simulink model "Pacemaker_Group1_1"  (R2020a)
settings: Solver=FixedStepAuto  StartTime=0.0  StopTime=10.0  FixedStep=1e-3  RelTol=1e-3  EnableMultiTasking=on
undefined symbols (not defined in the file): D0, D1, D10, D11, D12, D13, D2, D3, D4, D5, D6, D7, D8, D9, PTA0, PTA1, PTA2, PTB23, PTB9, PTC16, PTC17, PTC2, PTC3, PTC4, PTD0, PTD1, PTD2, PTD3
libraries: frdmk64flib x17
settings Model: SimulationMode=external  ExtModeTrigDuration=5  Creator=Luis  LastModifiedBy=jordanbierbrier
settings OptimizationCC: EnhancedBackFolding=on  PassReuseOutputArgsAs=Individual arguments  ZeroExternalMemoryAtStartup=off  ZeroInternalMemoryAtStartup=off  MaxStackSize=64  OptimizeBlockOrder=speed  DifferentSizesBufferReuse=on  OptimizationCustomize=off  EfficientTunableParamExpr=on
settings DebuggingCC: ParameterTunabilityLossMsg=error
settings HardwareCC: ProdBitPerPointer=32  ProdBitPerSizeT=32  ProdBitPerPtrDiffT=32  ProdLargestAtomicInteger=Long  ProdLargestAtomicFloat=Double  ProdWordSize=32  ProdHWDeviceType=ARM Compatible->ARM Cortex
settings SFSimCC: MATLABDynamicMemAlloc=off
settings RTWCC: SystemTargetFile=ert.tlc  HardwareBoard=NXP FRDM-K64F  TemplateMakefile=ert_default_tmf  Toolchain=GNU Tools for ARM Embedded Processors
settings CodeAppCC: ForceParamTrailComments=on  IgnoreCustomStorageClasses=off  OperatorAnnotations=on  SimulinkDataObjDesc=on  SFDataObjDesc=on  InsertBlockDesc=on
settings ERTTargetCC: ExtMode=on  ExtModeTransport=4  ExtModeMexFile=sendToCommService  ExtModeMexArgs='Pacemaker_Group1' 0

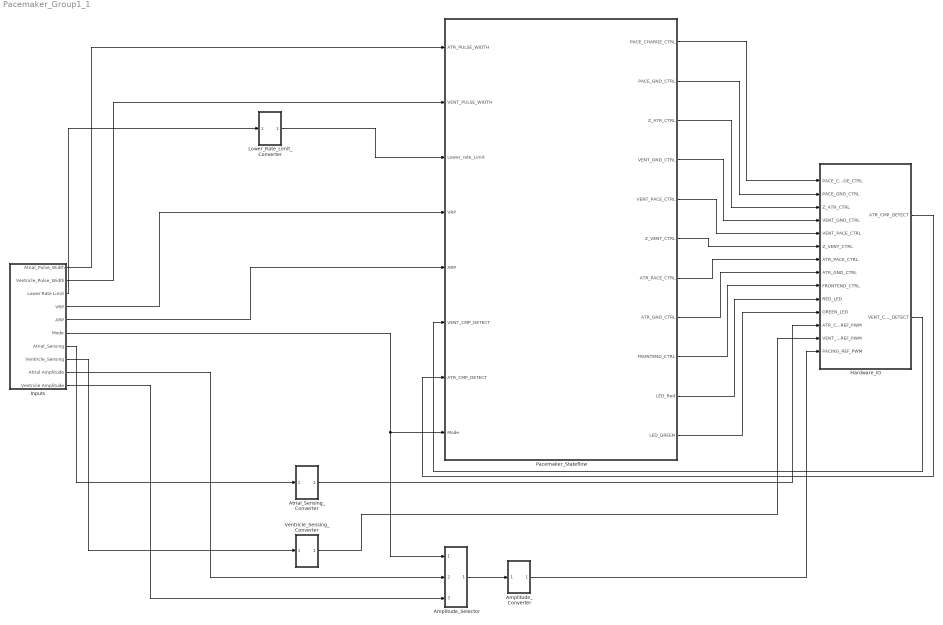
== system Pacemaker_Group1_1 ==
  Amplitude_Converter : Subsystem
  Amplitude_Selector : Subsystem
  Atrial_Sensing_Converter : Subsystem
  Hardware_IO : Subsystem
  Inputs : Subsystem
  Lower_Rate_Limit_Converter : Subsystem
  "Pacemaker_Stateflow " : Stateflow chart  TreatAsAtomicUnit=on
      settings: PortSchema="{\"entries\":[{\"content\":{\"sides\":[{\"content\":{\"connectorIds\":[\"In1\",\"In4\",\"In2\",\"In5\",\"In6\",\"In7\",\"In8\",\"In3\"]},\"type\":\"ConnectorPlacement.EquallySpacedRectSide\",\"uuid\":\"f97b12ff-cb00-4386-a373-7143c3a8b48d\"},{\"content\":{\"connectorIds\":[\"Out1\",\"Out2\",\"Out3\",\"Out4\",\"Out5\",\"Out6\",\"Out7\",\"Out8\",\"Out9\",\"Out10\",\"Out11\"],\"side\":\"RIGHT\"},\"type\":\"ConnectorPlacement.EquallySpacedRectSide\",\"uuid\":\"90163773-f9d1-46de-bd72-9589b8539202\"},{\"content\":{\"connectorIds\":[],\"side\":\"TOP\"},\"type\":\"ConnectorPlacement.EquallySpacedRectSide\",\"uuid\":\"f8a54119-a7c4-4071-8260-df405210e670\"},{\"content\":{\"connectorIds\":[],\"side\":\"BOTTOM\"},\"type\":\"ConnectorPlacement.EquallySpacedRectSide\",\"uuid\":\"70f9d800-d0b8-46e1-812e-9f4712f7acbd\"}]},\"type\":\"ConnectorPlacement.EquallySpacedConnector\",\"uuid\":\"47f7c40c-c42b-42f7-beed-99d299c6cdee\"}],\"packageUris\":[\"http://schema.mathworks.com/mf0/Connector/19700101\"],\"version\":\"1.0\"}"
  Ventricle_Sensing_Converter : Subsystem
  wires:
  Lower_Rate_Limit_Converter/1(Out1) -> "Pacemaker_Stateflow "/2(Lower_rate_Limit)
  Amplitude_Selector/1(Out1) -> Amplitude_Converter/1(In1)
  "Pacemaker_Stateflow "/1(PACE_CHARGE_CTRL) -> Hardware_IO/1(PACE_CHARGE_CTRL)
  "Pacemaker_Stateflow "/2(PACE_GND_CTRL) -> Hardware_IO/2(PACE_GND_CTRL)
  "Pacemaker_Stateflow "/3(Z_ATR_CTRL) -> Hardware_IO/3(Z_ATR_CTRL)
  "Pacemaker_Stateflow "/4(VENT_GND_CTRL) -> Hardware_IO/4(VENT_GND_CTRL)
  "Pacemaker_Stateflow "/5(VENT_PACE_CTRL) -> Hardware_IO/5(VENT_PACE_CTRL)
  "Pacemaker_Stateflow "/6(Z_VENT_CTRL) -> Hardware_IO/6(Z_VENT_CTRL)
  "Pacemaker_Stateflow "/7(ATR_PACE_CTRL) -> Hardware_IO/7(ATR_PACE_CTRL)
  "Pacemaker_Stateflow "/8(ATR_GND_CTRL) -> Hardware_IO/8(ATR_GND_CTRL)
  "Pacemaker_Stateflow "/9(FRONTEND_CTRL) -> Hardware_IO/9(FRONTEND_CTRL)
  "Pacemaker_Stateflow "/10(LED_Red) -> Hardware_IO/10(RED_LED)
  "Pacemaker_Stateflow "/11(LED_GREEN) -> Hardware_IO/11(GREEN_LED)
  Ventricle_Sensing_Converter/1(Out1) -> Hardware_IO/13(VENT_CMP_REF_PWM)
  Amplitude_Converter/1(Out1) -> Hardware_IO/14(PACING_REF_PWM)
  Hardware_IO/1(ATR_CMP_DETECT) -> "Pacemaker_Stateflow "/8(ATR_CMP_DETECT)
  Hardware_IO/2(VENT_CMP_DETECT) -> "Pacemaker_Stateflow "/7(VENT_CMP_DETECT)
  Atrial_Sensing_Converter/1(Out1) -> Hardware_IO/12(ATR_CMP_REF_PWM)
  Inputs/6(Mode) -> Amplitude_Selector/1(In1), "Pacemaker_Stateflow "/3(Mode)
  Inputs/1(Atrial_Pulse_Width) -> "Pacemaker_Stateflow "/1(ATR_PULSE_WIDTH)
  Inputs/2(Ventricle_Pulse_Width) -> "Pacemaker_Stateflow "/4(VENT_PULSE_WIDTH)
  Inputs/3(Lower Rate Limit) -> Lower_Rate_Limit_Converter/1(In1)
  Inputs/4(VRP) -> "Pacemaker_Stateflow "/5(VRP)
  Inputs/5(ARP) -> "Pacemaker_Stateflow "/6(ARP)
  Inputs/7(Atrial_Sensing) -> Atrial_Sensing_Converter/1(In1)
  Inputs/8(Ventricle_Sensing) -> Ventricle_Sensing_Converter/1(In1)
  Inputs/9(Atrial Amplitude) -> Amplitude_Selector/2(In2)
  Inputs/10(Ventricle Amplitude) -> Amplitude_Selector/3(In3)

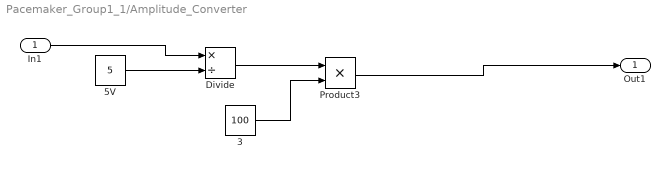
== system Pacemaker_Group1_1/Amplitude_Converter ==
  In1 : Inport
  3 : Constant  Value=100  OutDataTypeStr=double
  5V : Constant  Value=5  OutDataTypeStr=double
  Divide : Product  Inputs=*/  OutDataTypeStr=double  RndMeth=Nearest
  Product3 : Product  OutDataTypeStr=double
  Out1 : Outport
  wires:
  Product3/1 -> Out1/1
  3/1 -> Product3/2
  In1/1 -> Divide/1
  Divide/1 -> Product3/1
  5V/1 -> Divide/2

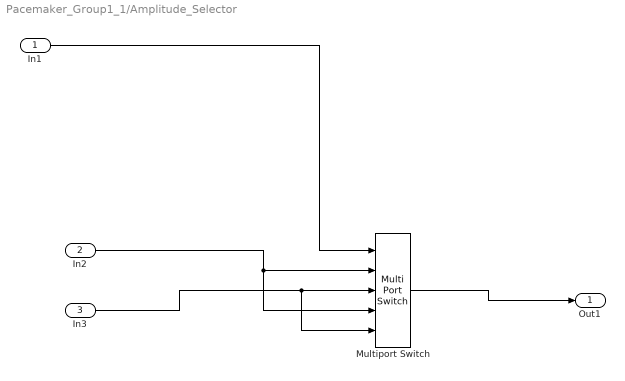
== system Pacemaker_Group1_1/Amplitude_Selector ==
  In1 : Inport
  In2 : Inport  Port=2
  In3 : Inport  Port=3
  Multiport Switch : MultiPortSwitch  DataPortOrder=Zero-based contiguous  Inputs=4  zeroidx=on  OutDataTypeStr=double
  Out1 : Outport
  wires:
  Multiport Switch/1 -> Out1/1
  In3/1 -> Multiport Switch/5, Multiport Switch/3
  In1/1 -> Multiport Switch/1
  In2/1 -> Multiport Switch/4, Multiport Switch/2

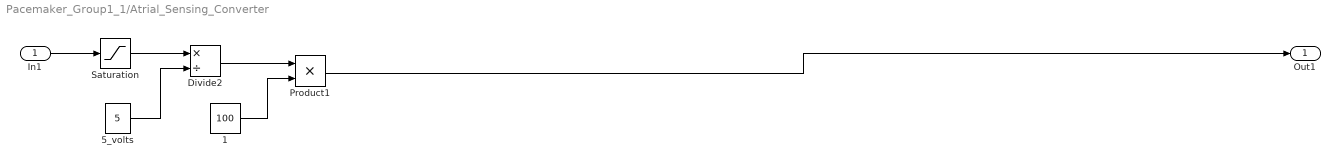
== system Pacemaker_Group1_1/Atrial_Sensing_Converter ==
  In1 : Inport
  1 : Constant  Value=100  OutDataTypeStr=uint16
  5_volts : Constant  Value=5  OutDataTypeStr=double
  Divide2 : Product  Inputs=*/
  Product1 : Product  OutDataTypeStr=uint16
  Saturation : Saturate  UpperLimit=4  LowerLimit=0.65  LinearizeAsGain=off  OutDataTypeStr=double
  Out1 : Outport
  wires:
  Product1/1 -> Out1/1
  1/1 -> Product1/2
  Divide2/1 -> Product1/1
  5_volts/1 -> Divide2/2
  In1/1 -> Saturation/1
  Saturation/1 -> Divide2/1

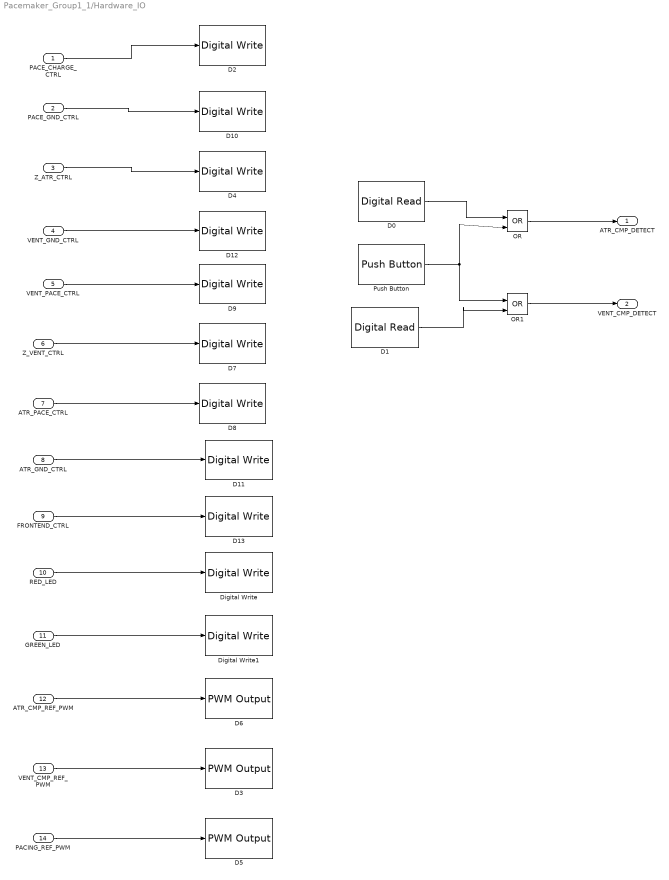
== system Pacemaker_Group1_1/Hardware_IO ==
  PACE_CHARGE_CTRL : Inport
  PACE_GND_CTRL : Inport  Port=2
  Z_ATR_CTRL : Inport  Port=3
  VENT_GND_CTRL : Inport  Port=4
  VENT_PACE_CTRL : Inport  Port=5
  Z_VENT_CTRL : Inport  Port=6
  ATR_PACE_CTRL : Inport  Port=7
  ATR_GND_CTRL : Inport  Port=8
  FRONTEND_CTRL : Inport  Port=9
  RED_LED : Inport  Port=10
  GREEN_LED : Inport  Port=11
  ATR_CMP_REF_PWM : Inport  Port=12
  VENT_CMP_REF_PWM : Inport  Port=13
  PACING_REF_PWM : Inport  Port=14
  D0 : frdmk64flib/Digital Read  Whichpin=PTC16 (D0)  SampleTime=-1
  D1 : frdmk64flib/Digital Read  Whichpin=PTC17 (D1)  SampleTime=-1
  D10 : frdmk64flib/Digital Write  Whichpin=PTD0 (D10)
  D11 : frdmk64flib/Digital Write  Whichpin=PTD2 (D11)
  D12 : frdmk64flib/Digital Write  Whichpin=PTD3 (D12)
  D13 : frdmk64flib/Digital Write  Whichpin=PTD1 (D13)
  D2 : frdmk64flib/Digital Write  Whichpin=PTB9 (D2)
  D3 : frdmk64flib/PWM Output  Whichpin=PTA1 (D3)  InitialFrequency=2000  InitialDutyCycle=0
  D4 : frdmk64flib/Digital Write  Whichpin=PTB23 (D4)
  D5 : frdmk64flib/PWM Output  Whichpin=PTA2 (D5)  InitialFrequency=2000  InitialDutyCycle=0
  D6 : frdmk64flib/PWM Output  Whichpin=PTC2 (D6)  InitialFrequency=2000  InitialDutyCycle=0
  D7 : frdmk64flib/Digital Write  Whichpin=PTC3 (D7)
  D8 : frdmk64flib/Digital Write  Whichpin=PTA0 (D8)
  D9 : frdmk64flib/Digital Write  Whichpin=PTC4 (D9)
  Digital Write : frdmk64flib/Digital Write  Whichpin=RED_LED
  Digital Write1 : frdmk64flib/Digital Write  Whichpin=GREEN_LED
  OR : Logic  Operator=OR  IconShape=distinctive  AllPortsSameDT=off  OutDataTypeStr=boolean
  OR1 : Logic  Operator=OR  IconShape=distinctive  AllPortsSameDT=off  OutDataTypeStr=boolean
  Push Button : frdmk64flib/Push Button  Whichswitch=SW2  SampleTime1=-1
  ATR_CMP_DETECT : Outport
  VENT_CMP_DETECT : Outport  Port=2
  wires:
  PACING_REF_PWM/1 -> D5/1
  RED_LED/1 -> Digital Write/1
  Z_ATR_CTRL/1 -> D4/1
  PACE_CHARGE_CTRL/1 -> D2/1
  VENT_GND_CTRL/1 -> D12/1
  D1/1 -> OR1/2
  ATR_PACE_CTRL/1 -> D8/1
  OR1/1 -> VENT_CMP_DETECT/1
  PACE_GND_CTRL/1 -> D10/1
  ATR_GND_CTRL/1 -> D11/1
  OR/1 -> ATR_CMP_DETECT/1
  D0/1 -> OR/1
  ATR_CMP_REF_PWM/1 -> D6/1
  Push Button/1 -> OR1/1, OR/2
  GREEN_LED/1 -> Digital Write1/1
  FRONTEND_CTRL/1 -> D13/1
  VENT_CMP_REF_PWM/1 -> D3/1
  Z_VENT_CTRL/1 -> D7/1
  VENT_PACE_CTRL/1 -> D9/1

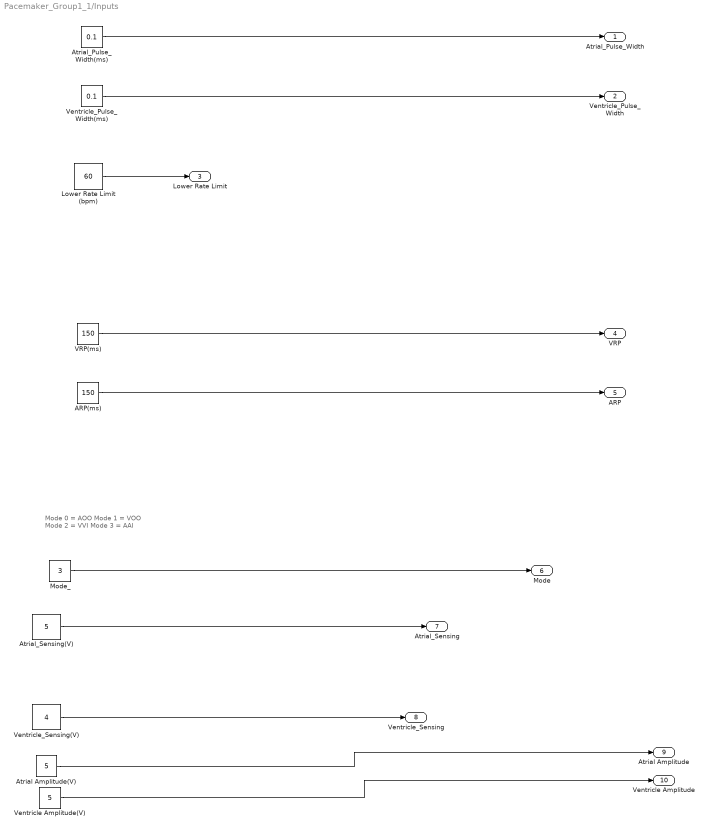
== system Pacemaker_Group1_1/Inputs ==
  note: Mode 0 = AOO
      | Mode 1 = VOO
      | Mode 2 = VVI
      | Mode 3 = AAI
  ARP(ms) : Constant  Value=150  OutDataTypeStr=uint16
  Atrial Amplitude(V) : Constant  Value=5  OutDataTypeStr=double
  Atrial_Pulse_Width(ms) : Constant  Value=0.1  OutDataTypeStr=double
  Atrial_Sensing(V) : Constant  Value=5  OutDataTypeStr=double
  Lower Rate Limit (bpm) : Constant  Value=60  OutDataTypeStr=uint16
  Mode_ : Constant  Value=3  OutDataTypeStr=double
  VRP(ms) : Constant  Value=150  OutDataTypeStr=uint16
  Ventricle Amplitude(V) : Constant  Value=5  OutDataTypeStr=double
  Ventricle_Pulse_Width(ms) : Constant  Value=0.1  OutDataTypeStr=double
  Ventricle_Sensing(V) : Constant  Value=4  OutDataTypeStr=double
  Atrial_Pulse_Width : Outport
  Ventricle_Pulse_Width : Outport  Port=2
  Lower Rate Limit : Outport  Port=3
  VRP : Outport  Port=4
  ARP : Outport  Port=5
  Mode : Outport  Port=6
  Atrial_Sensing : Outport  Port=7
  Ventricle_Sensing : Outport  Port=8
  Atrial Amplitude : Outport  Port=9
  Ventricle Amplitude : Outport  Port=10
  wires:
  Ventricle Amplitude(V)/1 -> Ventricle Amplitude/1
  Mode_/1 -> Mode/1
  Atrial_Sensing(V)/1 -> Atrial_Sensing/1
  ARP(ms)/1 -> ARP/1
  Atrial Amplitude(V)/1 -> Atrial Amplitude/1
  VRP(ms)/1 -> VRP/1
  Ventricle_Sensing(V)/1 -> Ventricle_Sensing/1
  Lower Rate Limit (bpm)/1 -> Lower Rate Limit/1
  Atrial_Pulse_Width(ms)/1 -> Atrial_Pulse_Width/1
  Ventricle_Pulse_Width(ms)/1 -> Ventricle_Pulse_Width/1

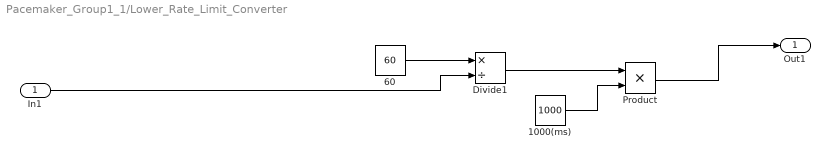
== system Pacemaker_Group1_1/Lower_Rate_Limit_Converter ==
  In1 : Inport
  1000(ms) : Constant  Value=1000  OutDataTypeStr=uint16
  60 : Constant  Value=60  OutDataTypeStr=uint16
  Divide1 : Product  Inputs=*/
  Product : Product  OutDataTypeStr=uint16
  Out1 : Outport
  wires:
  60/1 -> Divide1/1
  In1/1 -> Divide1/2
  Product/1 -> Out1/1
  Divide1/1 -> Product/1
  1000(ms)/1 -> Product/2

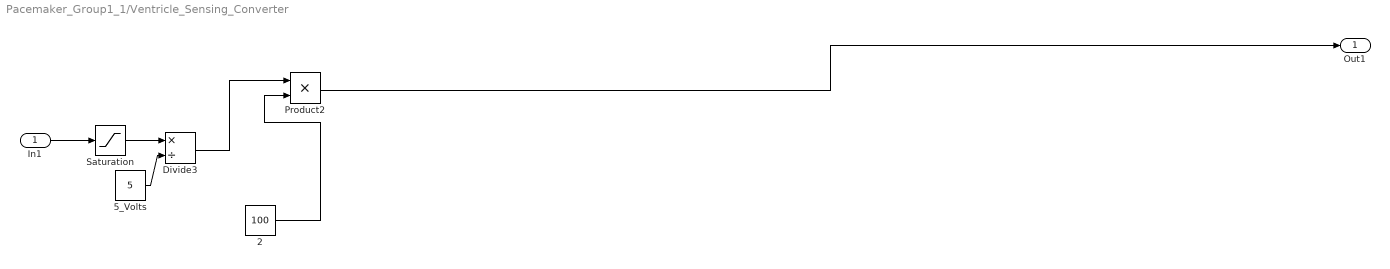
== system Pacemaker_Group1_1/Ventricle_Sensing_Converter ==
  In1 : Inport
  2 : Constant  Value=100  OutDataTypeStr=uint16
  5_Volts : Constant  Value=5  OutDataTypeStr=double
  Divide3 : Product  Inputs=*/
  Product2 : Product  OutDataTypeStr=uint16
  Saturation : Saturate  UpperLimit=4  LowerLimit=0.65  OutDataTypeStr=double
  Out1 : Outport
  wires:
  Product2/1 -> Out1/1
  5_Volts/1 -> Divide3/2
  Divide3/1 -> Product2/1
  In1/1 -> Saturation/1
  2/1 -> Product2/2
  Saturation/1 -> Divide3/1

== stateflow chart Pacemaker_Group1_1/Pacemaker_Stateflow  ==
  state AOO
    state AOO_CHARGING
      entry:
      %Charge C22
      ATR_PACE_CTRL=false;
      VENT_PACE_CTRL=false;
      PACE_CHARGE_CTRL=true;
      %Discharge C21
      PACE_GND_CTRL=true;
      Z_VENT_CTRL=false;
      Z_ATR_CTRL=false;
      ATR_GND_CTRL=true;
      VENT_GND_CTRL=false;
      LED_Red = false;
    state AOO_DISCHARGING
      entry:
      %Discharge C22 into ATR
      %Charge C21
      PACE_CHARGE_CTRL=false;
      PACE_GND_CTRL=true;
      ATR_PACE_CTRL=true;
      ATR_GND_CTRL=false;
      Z_VENT_CTRL=false;
      Z_ATR_CTRL=false;
      VENT_GND_CTRL=false;
      VENT_PACE_CTRL=false;
      LED_Red = true;
    AOO_DISCHARGING -> AOO_CHARGING : after(ATR_PULSE_WIDTH,msec)
    AOO_CHARGING -> AOO_DISCHARGING : after(Lower_rate_Limit - ATR_PULSE_WIDTH,msec)
  state VOO [group]
    state VOO_CHARGING
      entry:
      %Charge C22
      VENT_PACE_CTRL=false;
      ATR_PACE_CTRL=false;
      PACE_CHARGE_CTRL=true;
      %Discharge C21
      PACE_GND_CTRL=true;
      Z_VENT_CTRL=false;
      Z_ATR_CTRL=false;
      ATR_PACE_CTRL=false;
      ATR_GND_CTRL=false;
      VENT_GND_CTRL=true;
      LED_GREEN = false;
    state VOO_DISCHARGE
      entry:
      %Discharge C22 into VENT
      %Charge C21
      PACE_CHARGE_CTRL=false;
      PACE_GND_CTRL=true;
      ATR_PACE_CTRL=false;
      ATR_GND_CTRL=false;
      Z_ATR_CTRL=false
      Z_VENT_CTRL=false;
      VENT_GND_CTRL=false;
      VENT_PACE_CTRL=true;
      LED_GREEN = true;
    VOO_DISCHARGE -> VOO_CHARGING : after(VENT_PULSE_WIDTH, msec)
    VOO_CHARGING -> VOO_DISCHARGE : after(Lower_rate_Limit - VENT_PULSE_WIDTH, msec)
  state Intial_State
    entry:
    %Charge C22
    ATR_PACE_CTRL=false;
    VENT_PACE_CTRL=false;
    PACE_CHARGE_CTRL=false;
    %Discharge C21
    PACE_GND_CTRL=false;
    Z_VENT_CTRL=false;
    Z_ATR_CTRL=false;
    ATR_GND_CTRL=false;
    VENT_GND_CTRL=false;
  state VVI [group]
    state CHARGING_C22
      entry:
      FRONTEND_CTRL = true;
      PACE_GND_CTRL = true;
      VENT_PACE_CTRL=false;
      ATR_PACE_CTRL=false;
      PACE_CHARGE_CTRL=true;
      Z_VENT_CTRL=false;
      Z_ATR_CTRL=false;
      ATR_GND_CTRL=false;
      VENT_GND_CTRL=true;
      LED_GREEN = false;
    state VENTRICAL_PACE
      entry:
      FRONTEND_CTRL = false;
      PACE_GND_CTRL = true;
      VENT_PACE_CTRL=true;
      ATR_PACE_CTRL=false;
      PACE_CHARGE_CTRL=false;
      Z_VENT_CTRL=false;
      Z_ATR_CTRL=false;
      ATR_GND_CTRL=false;
      VENT_GND_CTRL=false;
      LED_GREEN = true;
    state VRP_State
      entry:
      PACE_GND_CTRL = true;
      VENT_PACE_CTRL=false;
      ATR_PACE_CTRL=false;
      PACE_CHARGE_CTRL=true;
      Z_VENT_CTRL=false;
      Z_ATR_CTRL=false;
      ATR_GND_CTRL=false;
      VENT_GND_CTRL=true;
      LED_GREEN = false;
    VVI.CHARGING_C22 -> VENTRICAL_PACE [order 2] : after((Lower_rate_Limit) - (VENT_PULSE_WIDTH + VRP), msec)
    VVI.CHARGING_C22 -> VRP_State [order 1] : [VENT_CMP_DETECT == true]
    VRP_State -> VVI.CHARGING_C22 : after(VRP, msec)
    VENTRICAL_PACE -> VRP_State : after(VENT_PULSE_WIDTH, msec)
  state AAI [group]
    state CHARGING_C22
      entry:
      FRONTEND_CTRL = true;
      PACE_GND_CTRL = true;
      VENT_PACE_CTRL=false;
      ATR_PACE_CTRL=false;
      PACE_CHARGE_CTRL=true;
      Z_VENT_CTRL=false;
      Z_ATR_CTRL=false;
      ATR_GND_CTRL=true;
      VENT_GND_CTRL=false;
      LED_Red = false;
    state ATRIAL_PACE
      entry:
      FRONTEND_CTRL = false;
      PACE_GND_CTRL = true;
      VENT_PACE_CTRL=false;
      ATR_PACE_CTRL=true;
      PACE_CHARGE_CTRL=false;
      Z_VENT_CTRL=false;
      Z_ATR_CTRL=false;
      ATR_GND_CTRL=false;
      VENT_GND_CTRL=false;
      LED_Red = true;
    state ARP_State
      entry:
      PACE_GND_CTRL = true;
      VENT_PACE_CTRL=false;
      ATR_PACE_CTRL=false;
      PACE_CHARGE_CTRL=true;
      Z_VENT_CTRL=false;
      Z_ATR_CTRL=false;
      ATR_GND_CTRL=true;
      VENT_GND_CTRL=false;
      LED_Red = false;
    AAI.CHARGING_C22 -> ATRIAL_PACE [order 2] : after((Lower_rate_Limit) - (ATR_PULSE_WIDTH + ARP), msec)
    AAI.CHARGING_C22 -> ARP_State [order 1] : [ATR_CMP_DETECT == true]
    ARP_State -> AAI.CHARGING_C22 : after(ARP, msec)
    ATRIAL_PACE -> ARP_State : after(ATR_PULSE_WIDTH, msec)
  Intial_State -> AOO_CHARGING [order 1] : [Mode == 0]
  Intial_State -> VOO_CHARGING [order 2] : [Mode == 1]
  (default) -> Intial_State
  Intial_State -> VVI.CHARGING_C22 [order 3] : [Mode == 2]
  Intial_State -> AAI.CHARGING_C22 [order 4] : [Mode == 3]
  data: PACE_CHARGE_CTRL output boolean; PACE_GND_CTRL output boolean; Z_ATR_CTRL output boolean; VENT_GND_CTRL output boolean; VENT_PACE_CTRL output boolean; Z_VENT_CTRL output boolean; ATR_PULSE_WIDTH input double; Lower_rate_Limit input uint16; Mode input double; ATR_PACE_CTRL output boolean; ATR_GND_CTRL output boolean; VENT_PULSE_WIDTH input double; VRP input uint16; ARP input uint16; FRONTEND_CTRL output boolean; VENT_CMP_DETECT input boolean; ATR_CMP_DETECT input boolean; LED_Red output boolean; LED_GREEN output boolean
